simulink model "qAjustePID_OUT"  (Simulink 7.7)
settings: Solver=FixedStepDiscrete  StartTime=0.0  StopTime=inf  FixedStep=0.2  RelTol=1e-3
libraries: simulink x6, aerolibanimutils x1
settings Model: Creator=claus  LastModifiedBy=claus

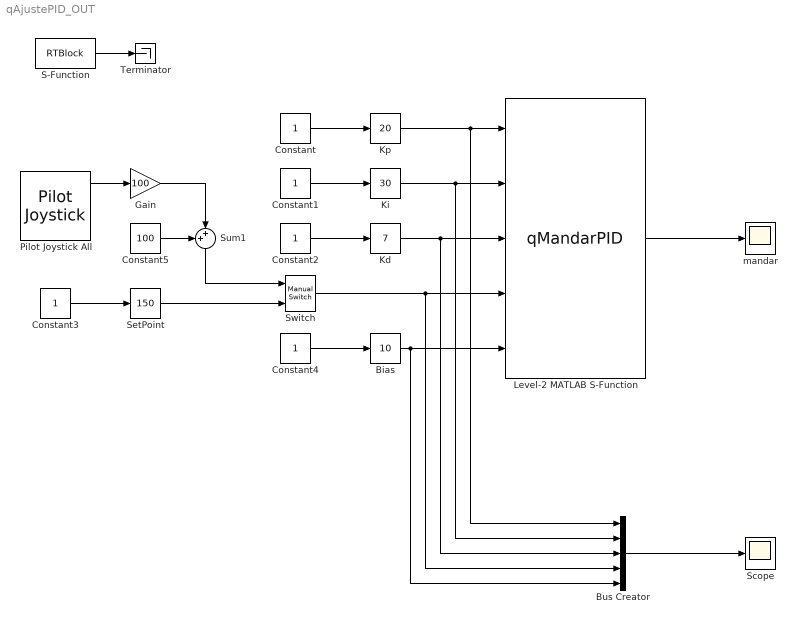
== system qAjustePID_OUT ==
  Bias : simulink/Math Operations/Slider Gain  SystemSampleTime=-1  low=0  gain=10  high=20
  Bus Creator : BusCreator  Inputs=5
  Constant{,1..4} (5 alike) : Constant
  Constant5 : Constant  Value=100
  Gain : Gain  Gain=100
  Kd : simulink/Math Operations/Slider Gain  SystemSampleTime=-1  low=0  gain=7  high=20
  Ki : simulink/Math Operations/Slider Gain  SystemSampleTime=-1  low=0  gain=30  high=50
  Kp : simulink/Math Operations/Slider Gain  SystemSampleTime=-1  low=0  gain=20  high=20
  Level-2 MATLAB S-Function : M-S-Function  FunctionName=qMandarPID  Parameters=host, puerto  mask(mandarPID){host='192.168.1.8', puerto=58887}
      mask prompts: host "Host (o 1 mostrar por consola)"
      mask help:
      | Manda los 4 parámetros de un controlador PID a través de un socket a un servidor corriendo en host:puerto.
      | Para mostrar la salida por la consola poner 1 en host.
      | El formato de salida se especifica en qFormatearPID_OUT.m
      mask Display:
      | port_label('input', 1, 'Kp');
      | port_label('input', 2, 'Ki');
      | port_label('input', 3, 'Kd');
      | port_label('input', 4, 'SetPoing');
      | port_label('input', 5, 'Bias');
      | port_label('output', 1, 'Mandar');
      | 
      | fprintf('qMandarPID');
  Pilot Joystick All : aerolibanimutils/Pilot Joystick  JoystickID=Joystick1  OutputConfiguration=FourAxis  SampleTime=-1
  S-Function : S-Function  FunctionName=RTBlock  Parameters=50, 'HIGH', 'TIME CRITICAL'  EnableBusSupport=off
  Scope : Scope
      settings: TimeRange=10  YMin=0  YMax=200
  SetPoint : simulink/Math Operations/Slider Gain  SystemSampleTime=-1  low=0  gain=150  high=500
  Sum1 : Sum  Inputs=++|
  Switch : simulink/Signal Routing/Manual Switch  SystemSampleTime=-1  sw=0  action=0  varsize=off
  Terminator : Terminator
  mandar : Scope
      settings: TimeRange=10  YMin=0  YMax=200
  wires:
  Constant/1 -> Kp/1
  Kp/1 -> Level-2 MATLAB S-Function/1, Bus Creator/1
  Constant1/1 -> Ki/1
  Ki/1 -> Level-2 MATLAB S-Function/2, Bus Creator/2
  Constant2/1 -> Kd/1
  Kd/1 -> Level-2 MATLAB S-Function/3, Bus Creator/3
  Bus Creator/1 -> Scope/1
  S-Function/1 -> Terminator/1
  Constant4/1 -> Bias/1
  Bias/1 -> Level-2 MATLAB S-Function/5, Bus Creator/5
  Switch/1 -> Level-2 MATLAB S-Function/4, Bus Creator/4
  Constant3/1 -> SetPoint/1
  SetPoint/1 -> Switch/2
  Pilot Joystick All/1 -> Gain/1
  Gain/1 -> Sum1/2
  Sum1/1 -> Switch/1
  Constant5/1 -> Sum1/1
  Level-2 MATLAB S-Function/1 -> mandar/1
